simulink model "SMA_Wire_Controller"  (R2023b)
settings: Solver=FixedStepAuto  StartTime=0  StopTime=2  FixedStep=0.00001  RelTol=1e-5  EnableMultiTasking=on
values from neighbouring files (symbols this model uses):
  Da = 75.0e9    (= 75000000000)    [SMA_Initialize.m]
  Dm = 28.0e9    (= 28000000000)    [SMA_Initialize.m]
  epsR = 0.04    [SMA_Initialize.m]
  HeatCap = 837.3    [SMA_Initialize.m]
  HeatTransCoeff = 150    [SMA_Initialize.m]
  Inertia = 0.5*PullyMass*PullyRadius^2*0.001    (= 1e-08)    [SMA_Initialize.m]
  Length = 0.5    [SMA_Initialize.m]
  pa = 100*10^-8    (= 1e-06)    [SMA_Initialize.m]
  pm = 80*10^-8    (= 8e-07)    [SMA_Initialize.m]
  PullyRadius = 0.02    [SMA_Initialize.m]
  SectA = pi*(Diameter^2)/4    (= 3.14159265359e-08)    [SMA_Initialize.m]
  SurfArea = Diameter*Length*pi    (= 0.000314159265359)    [SMA_Initialize.m]
  TempAmb = 25    [SMA_Initialize.m]
  thetaT = 0    [SMA_Initialize.m]
  WireMass = (Density*pi*(Diameter^2)*Length)/4    (= 0.000101316363078)    [SMA_Initialize.m]
libraries: simulink x2
settings Model: Creator=Jack  LastModifiedBy=Jack
settings SolverCC: ZeroCrossControl=EnableAll  ZeroCrossAlgorithm=Adaptive
settings DebuggingCC: SignalInfNanChecking=error  ParameterPrecisionLossMsg=none
settings HardwareCC: ProdBitPerLong=64  ProdLargestAtomicFloat=Double  ProdHWDeviceType=AMD->Athlon 64

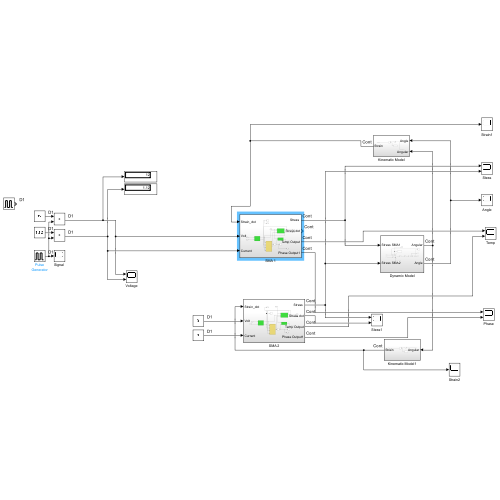
[thumbnail: Simulink's stored preview of the top-level diagram]
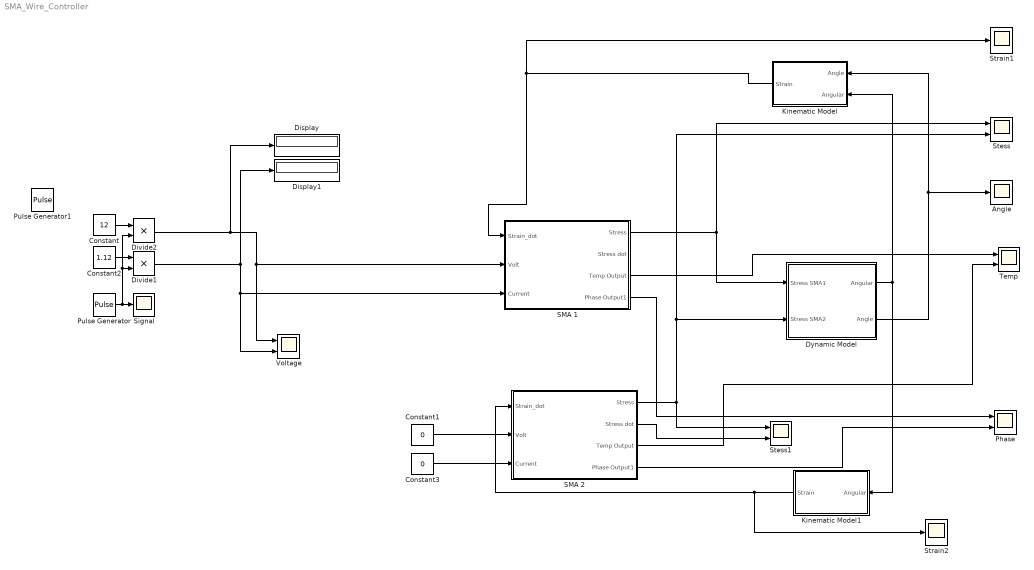
== system SMA_Wire_Controller ==
  Angle : Scope
  Constant : Constant  Value=12  SampleTime=0.00001
  Constant1 : Constant  Value=0  SampleTime=0.00001
  Constant2 : Constant  Value=1.12  SampleTime=0.00001
  Constant3 : Constant  Value=0  SampleTime=0.00001
  Display : Display
  Display1 : Display
  Divide1 : Product  Inputs=**
  Divide2 : Product  Inputs=**
  Dynamic Model : Subsystem
  Kinematic Model : Subsystem
  Kinematic Model1 : Subsystem
  Phase : Scope  NumInputPorts=2
  Pulse Generator : DiscretePulseGenerator  PulseType=Time based  Period=40  PulseWidth=1.5  PhaseDelay=0.25
  Pulse Generator1 : DiscretePulseGenerator  PulseType=Time based  Amplitude=0.5  Period=10  PulseWidth=5
  SMA 1 : Subsystem
  SMA 2 : Subsystem
  "Signal " : Scope
  Stess : Scope  NumInputPorts=2
  Stess1 : Scope  NumInputPorts=2
  Strain1 : Scope
  Strain2 : Scope
  Temp : Scope  NumInputPorts=2
  Voltage : Scope  NumInputPorts=2
  wires:
  Divide2/1 -> SMA 1/2(Volt), Voltage/1, Display/1
  Pulse Generator/1 -> Divide1/2, Divide2/2, "Signal "/1
  Divide1/1 -> Voltage/2, SMA 1/3(Current), Display1/1
  Dynamic Model/2(Angle) -> Kinematic Model/1(Angle), Angle/1
  Constant/1 -> Divide2/1
  Constant2/1 -> Divide1/1
  Kinematic Model/1(Strain) -> SMA 1/1(Strain_dot), Strain1/1
  Dynamic Model/1(Angular) -> Kinematic Model/2(Angular), Kinematic Model1/1(Angular)
  SMA 1/1("Stress ") -> Dynamic Model/1(Stress SMA1), Stess/1
  Kinematic Model1/1(Strain) -> Strain2/1, SMA 2/1(Strain_dot)
  SMA 2/1("Stress ") -> Stess1/1, Dynamic Model/2(Stress SMA2), Stess/2
  SMA 2/2(Stress dot) -> Stess1/2
  SMA 1/3(Temp Output) -> Temp/1
  SMA 2/3(Temp Output) -> Temp/2
  SMA 1/4(Phase Output1) -> Phase/1
  SMA 2/4(Phase Output1) -> Phase/2
  Constant1/1 -> SMA 2/2(Volt)
  Constant3/1 -> SMA 2/3(Current)

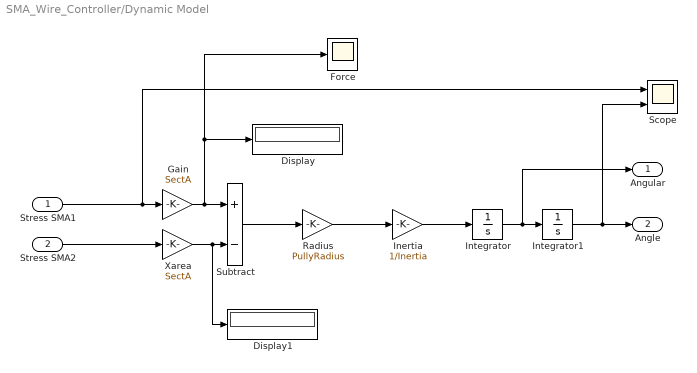
== system SMA_Wire_Controller/Dynamic Model ==
  Stress SMA1 : Inport
  Stress SMA2 : Inport  Port=2
  Display : Display
  Display1 : Display
  Force : Scope
  Gain : Gain  Gain=SectA
  Inertia : Gain  Gain=1/Inertia
  Integrator : Integrator
  Integrator1 : Integrator
  Radius : Gain  Gain=PullyRadius
  Scope : Scope  NumInputPorts=2
  Subtract : Sum  Inputs=+-
  Xarea : Gain  Gain=SectA  OutDataTypeStr=single
  Angular : Outport
  Angle : Outport  Port=2
  wires:
  Gain/1 -> Subtract/1, Display/1, Force/1
  Xarea/1 -> Display1/1, Subtract/2
  Subtract/1 -> Radius/1
  Radius/1 -> Inertia/1
  Inertia/1 -> Integrator/1
  Integrator/1 -> Angular/1, Integrator1/1
  Stress SMA1/1 -> Scope/1, Gain/1
  Stress SMA2/1 -> Xarea/1
  Integrator1/1 -> Angle/1, Scope/2

== system SMA_Wire_Controller/Kinematic Model ==
  Angle : Inport
  Angular : Inport  Port=2
  -r : Gain  Gain=-PullyRadius
  Constant : Constant  Value=Length  SampleTime=0.00001
  Divide : Product  Inputs=*/
  Strain : Outport
  wires:
  Constant/1 -> Divide/2
  -r/1 -> Divide/1
  Angle/1 -> -r/1
  Divide/1 -> Strain/1

== system SMA_Wire_Controller/Kinematic Model1 ==
  Angular : Inport
  -r : Gain  Gain=PullyRadius
  Constant : Constant  Value=Length  SampleTime=0.00001
  Divide : Product  Inputs=*/
  Strain : Outport
  wires:
  Constant/1 -> Divide/2
  -r/1 -> Divide/1
  Angular/1 -> -r/1
  Divide/1 -> Strain/1

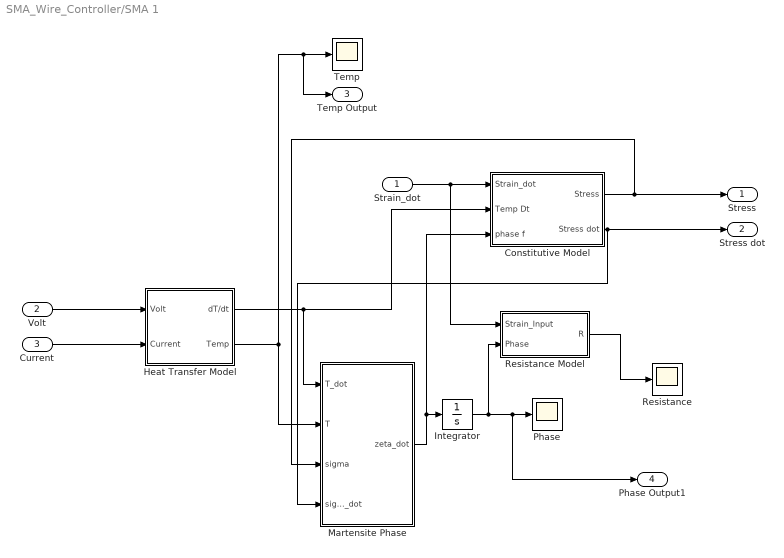
== system SMA_Wire_Controller/SMA 1 ==
  Strain_dot : Inport
  Volt : Inport  Port=2
  Current : Inport  Port=3
  Constitutive Model : Subsystem
  Heat Transfer Model : Subsystem
  Integrator : Integrator  InitialCondition=1
  "Martensite Phase " : Subsystem
  Phase : Scope
  Resistance : Scope
  Resistance Model : Subsystem
  Temp : Scope
  "Stress " : Outport
  Stress dot : Outport  Port=2
  Temp Output : Outport  Port=3
  Phase Output1 : Outport  Port=4
  wires:
  Current/1 -> Heat Transfer Model/2(Current)
  Resistance Model/1(R) -> Resistance/1
  Heat Transfer Model/1(dT/dt) -> "Martensite Phase "/1(T_dot), Constitutive Model/2(Temp Dt)
  "Martensite Phase "/1(zeta_dot) -> Constitutive Model/3(phase f), Integrator/1
  Volt/1 -> Heat Transfer Model/1(Volt)
  Strain_dot/1 -> Resistance Model/1(Strain_Input), Constitutive Model/1(Strain_dot)
  Heat Transfer Model/2(Temp) -> "Martensite Phase "/2(T), Temp Output/1, Temp/1
  Constitutive Model/1("Stress ") -> "Martensite Phase "/3(sigma), "Stress "/1
  Constitutive Model/2(Stress dot) -> "Martensite Phase "/4(sigma_dot), Stress dot/1
  Integrator/1 -> Resistance Model/2(Phase), Phase Output1/1, Phase/1

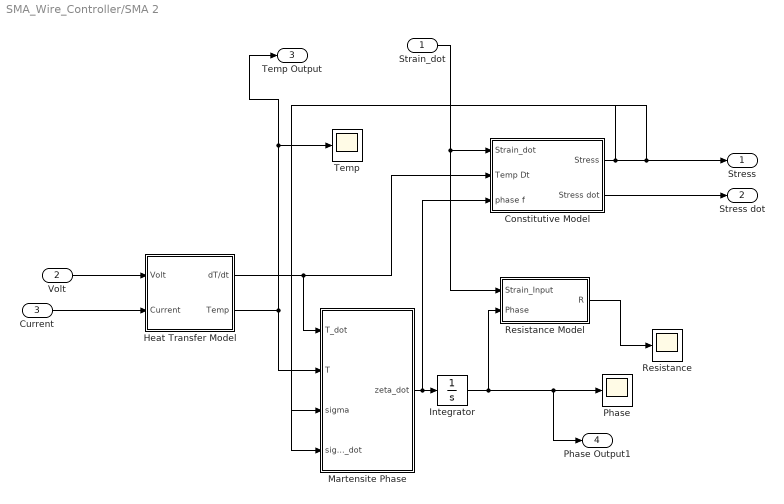
== system SMA_Wire_Controller/SMA 2 ==
  Strain_dot : Inport
  Volt : Inport  Port=2
  Current : Inport  Port=3
  Constitutive Model : Subsystem
  Heat Transfer Model : Subsystem
  Integrator : Integrator  InitialCondition=1
  "Martensite Phase " : Subsystem
  Phase : Scope
  Resistance : Scope
  Resistance Model : Subsystem
  Temp : Scope
  "Stress " : Outport
  Stress dot : Outport  Port=2
  Temp Output : Outport  Port=3
  Phase Output1 : Outport  Port=4
  wires:
  Current/1 -> Heat Transfer Model/2(Current)
  Resistance Model/1(R) -> Resistance/1
  Heat Transfer Model/1(dT/dt) -> "Martensite Phase "/1(T_dot), Constitutive Model/2(Temp Dt)
  Volt/1 -> Heat Transfer Model/1(Volt)
  Strain_dot/1 -> Resistance Model/1(Strain_Input), Constitutive Model/1(Strain_dot)
  Heat Transfer Model/2(Temp) -> "Martensite Phase "/2(T), Temp Output/1, Temp/1
  Constitutive Model/1("Stress ") -> "Martensite Phase "/3(sigma), "Martensite Phase "/4(sigma_dot), "Stress "/1
  Constitutive Model/2(Stress dot) -> Stress dot/1
  "Martensite Phase "/1(zeta_dot) -> Constitutive Model/3(phase f), Integrator/1
  Integrator/1 -> Resistance Model/2(Phase), Phase Output1/1, Phase/1

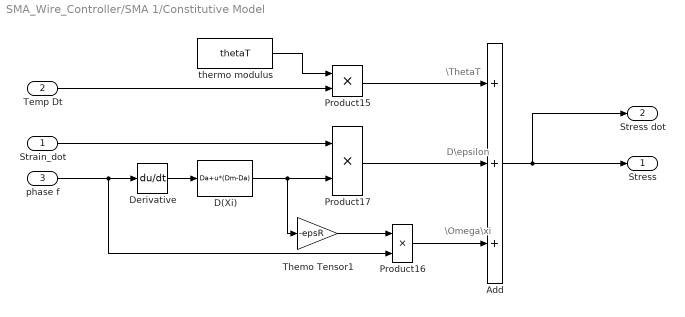
== system SMA_Wire_Controller/SMA 1/Constitutive Model ==
  note: \Omega\xi
  note: \ThetaT
  note: D\epsilon
  Strain_dot : Inport
  Temp Dt : Inport  Port=2
  phase f : Inport  Port=3
  Add : Sum  Inputs=+++
  D(Xi) : Fcn  Expr=Da+u*(Dm-Da)
  Derivative : Derivative
  Product15 : Product
  Product16 : Product
  Product17 : Product
  Themo Tensor1 : Gain  Gain=-epsR  SaturateOnIntegerOverflow=on  OutDataTypeStr=Inherit: Same as input  ParamDataTypeStr=Inherit: Same as input
  thermo modulus : Constant  Value=thetaT  SampleTime=0.00001
  "Stress " : Outport
  Stress dot : Outport  Port=2
  wires:
  Product15/1 -> Add/1
  Temp Dt/1 -> Product15/2
  thermo modulus/1 -> Product15/1
  D(Xi)/1 -> Product17/2, Themo Tensor1/1
  Themo Tensor1/1 -> Product16/1
  Add/1 -> "Stress "/1, Stress dot/1
  Product17/1 -> Add/2
  Product16/1 -> Add/3
  Strain_dot/1 -> Product17/1
  phase f/1 -> Derivative/1, Product16/2
  Derivative/1 -> D(Xi)/1

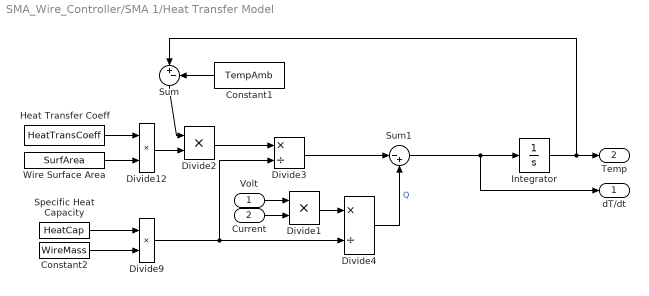
== system SMA_Wire_Controller/SMA 1/Heat Transfer Model ==
  Volt : Inport
  Current : Inport  Port=2
  Constant1 : Constant  Value=TempAmb  SampleTime=0.00001
  Constant2 : Constant  Value=WireMass  SampleTime=0.00001
  Divide{1..2,9,12} (4 alike) : Product  Inputs=**
  Divide3 : Product  Inputs=*/
  Divide4 : Product  Inputs=*/
  Heat Transfer Coeff : Constant  Value=HeatTransCoeff  SampleTime=0.00001
  Integrator : Integrator  InitialCondition=TempAmb
  Specific Heat Capacity : Constant  Value=HeatCap  SampleTime=0.00001
  Sum : Sum  Inputs=|+-
  Sum1 : Sum  Inputs=|-+
  Wire Surface Area : Constant  Value=SurfArea  SampleTime=0.00001
  dT/dt : Outport
  Temp : Outport  Port=2
  wires:
  Divide4/1 -> Sum1/2  "Q"
  Integrator/1 -> Temp/1, Sum/1
  Divide2/1 -> Divide3/1
  Heat Transfer Coeff/1 -> Divide12/1
  Divide9/1 -> Divide4/2, Divide3/2
  Constant1/1 -> Sum/2
  Wire Surface Area/1 -> Divide12/2
  Volt/1 -> Divide1/1
  Current/1 -> Divide1/2
  Divide12/1 -> Divide2/2
  Specific Heat Capacity/1 -> Divide9/1
  Divide1/1 -> Divide4/1
  Divide3/1 -> Sum1/1
  Sum/1 -> Divide2/1
  Sum1/1 -> dT/dt/1, Integrator/1
  Constant2/1 -> Divide9/2

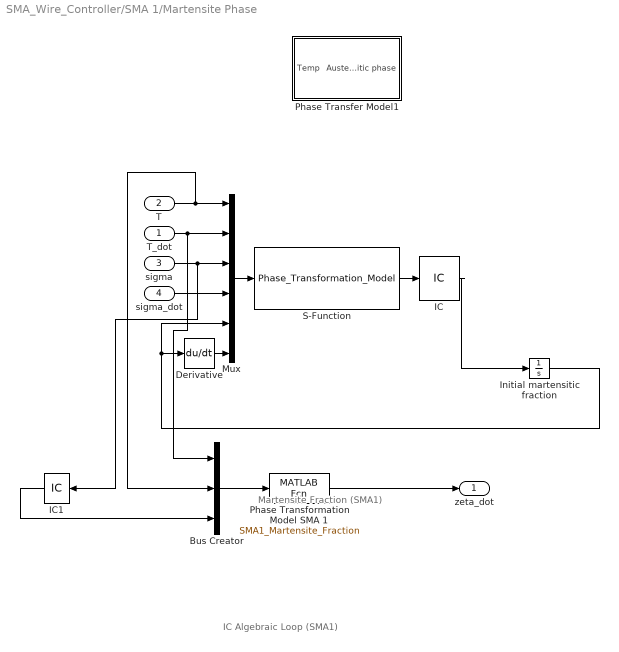
== system SMA_Wire_Controller/SMA 1/Martensite Phase  ==
  note: Martensite
      | Fraction (SMA1)
  note: IC Algebraic
      | Loop (SMA1)
  T_dot : Inport
  T : Inport  Port=2
  sigma : Inport  Port=3
  sigma_dot : Inport  Port=4
  Bus Creator : BusCreator  DialogController=Simulink.DDGSource_Bus  Inputs=3
  Derivative : Derivative
  IC : InitialCondition  Value=0
  IC1 : InitialCondition  Value=0
  Initial martensitic fraction : Integrator  InitialCondition=1  UpperSaturationLimit=1  LowerSaturationLimit=0
  Mux : Mux  Inputs=6
  Phase Transfer Model1 : Subsystem
  Phase Transformation Model SMA 1 : MATLABFcn  MATLABFcn=SMA1_Martensite_Fraction  OutputDimensions=1
  S-Function : S-Function  FunctionName=Phase_Transformation_Model  SFunctionDeploymentMode=off  EnableBusSupport=off
  zeta_dot : Outport
  wires:
  Initial martensitic fraction/1 -> Derivative/1, Mux/5
  Derivative/1 -> Mux/6
  S-Function/1 -> IC/1
  sigma_dot/1 -> Mux/4
  Mux/1 -> S-Function/1
  T/1 -> Bus Creator/2, Mux/1
  sigma/1 -> IC1/1, Mux/3
  T_dot/1 -> Bus Creator/1, Mux/2
  IC/1 -> Initial martensitic fraction/1
  IC1/1 -> Bus Creator/3
  Phase Transformation Model SMA 1/1 -> zeta_dot/1
  Bus Creator/1 -> Phase Transformation Model SMA 1/1

== system SMA_Wire_Controller/SMA 1/Resistance Model ==
  Strain_Input : Inport
  Phase : Inport  Port=2
  Constant : Constant
  Product : Product
  Product1 : Product
  Ra : Subsystem
  Rm : Subsystem
  Scope : Scope  NumInputPorts=2
  Subtract : Sum  Inputs=+-
  Sum : Sum  Inputs=|++
  R : Outport
  wires:
  Rm/1(Rm) -> Product/1
  Sum/1 -> R/1
  Product/1 -> Scope/1, Sum/1
  Constant/1 -> Subtract/1
  Phase/1 -> Subtract/2, Product/2
  Subtract/1 -> Product1/1
  Ra/1(Ra) -> Product1/2
  Product1/1 -> Sum/2, Scope/2
  Strain_Input/1 -> Ra/1(Strain), Rm/1(Strain)

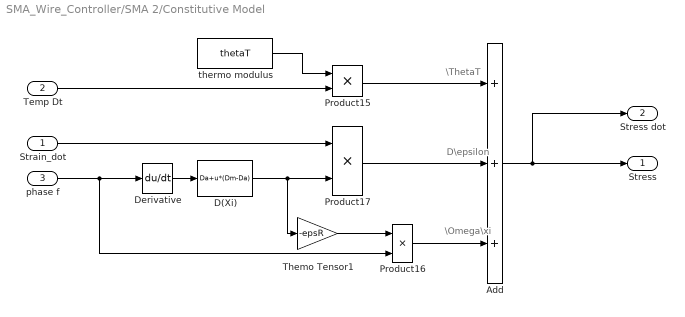
== system SMA_Wire_Controller/SMA 2/Constitutive Model ==
  note: \Omega\xi
  note: \ThetaT
  note: D\epsilon
  Strain_dot : Inport
  Temp Dt : Inport  Port=2
  phase f : Inport  Port=3
  Add : Sum  Inputs=+++
  D(Xi) : Fcn  Expr=Da+u*(Dm-Da)
  Derivative : Derivative
  Product15 : Product
  Product16 : Product
  Product17 : Product
  Themo Tensor1 : Gain  Gain=-epsR  SaturateOnIntegerOverflow=on  OutDataTypeStr=Inherit: Same as input  ParamDataTypeStr=Inherit: Same as input
  thermo modulus : Constant  Value=thetaT  SampleTime=0.00001
  "Stress " : Outport
  Stress dot : Outport  Port=2
  wires:
  Product15/1 -> Add/1
  Temp Dt/1 -> Product15/2
  thermo modulus/1 -> Product15/1
  D(Xi)/1 -> Product17/2, Themo Tensor1/1
  Themo Tensor1/1 -> Product16/1
  Add/1 -> "Stress "/1, Stress dot/1
  Product17/1 -> Add/2
  Product16/1 -> Add/3
  Strain_dot/1 -> Product17/1
  phase f/1 -> Derivative/1, Product16/2
  Derivative/1 -> D(Xi)/1

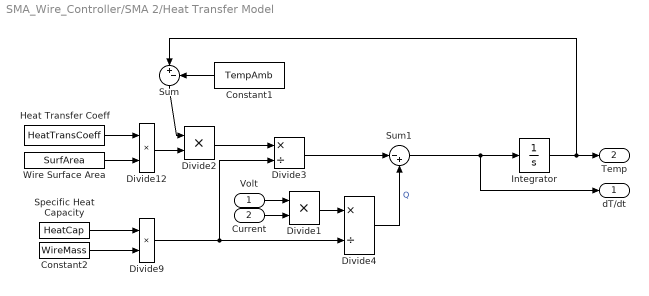
== system SMA_Wire_Controller/SMA 2/Heat Transfer Model ==
  Volt : Inport
  Current : Inport  Port=2
  Constant1 : Constant  Value=TempAmb  SampleTime=0.00001
  Constant2 : Constant  Value=WireMass  SampleTime=0.00001
  Divide{1..2,9,12} (4 alike) : Product  Inputs=**
  Divide3 : Product  Inputs=*/
  Divide4 : Product  Inputs=*/
  Heat Transfer Coeff : Constant  Value=HeatTransCoeff  SampleTime=0.00001
  Integrator : Integrator  InitialCondition=TempAmb
  Specific Heat Capacity : Constant  Value=HeatCap  SampleTime=0.00001
  Sum : Sum  Inputs=|+-
  Sum1 : Sum  Inputs=|-+
  Wire Surface Area : Constant  Value=SurfArea  SampleTime=0.00001
  dT/dt : Outport
  Temp : Outport  Port=2
  wires:
  Divide4/1 -> Sum1/2  "Q"
  Integrator/1 -> Temp/1, Sum/1
  Divide2/1 -> Divide3/1
  Heat Transfer Coeff/1 -> Divide12/1
  Divide9/1 -> Divide4/2, Divide3/2
  Constant1/1 -> Sum/2
  Wire Surface Area/1 -> Divide12/2
  Volt/1 -> Divide1/1
  Current/1 -> Divide1/2
  Divide12/1 -> Divide2/2
  Specific Heat Capacity/1 -> Divide9/1
  Divide1/1 -> Divide4/1
  Divide3/1 -> Sum1/1
  Sum/1 -> Divide2/1
  Sum1/1 -> dT/dt/1, Integrator/1
  Constant2/1 -> Divide9/2

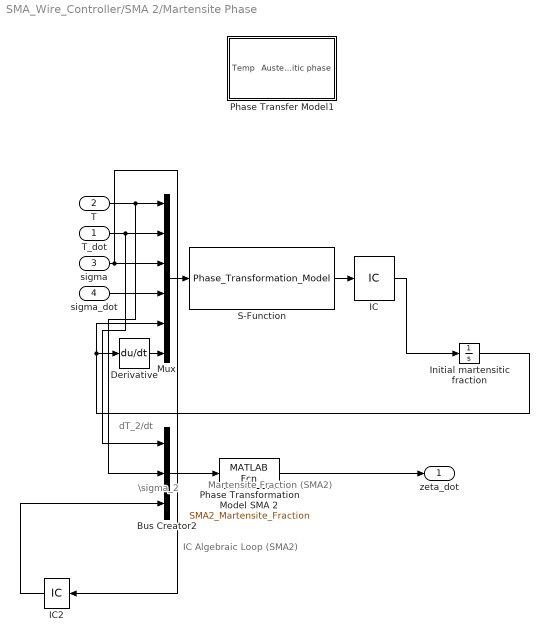
== system SMA_Wire_Controller/SMA 2/Martensite Phase  ==
  note: \sigma_2
  note: IC Algebraic
      | Loop (SMA2)
  note: Martensite
      | Fraction (SMA2)
  note: dT_2/dt
  T_dot : Inport
  T : Inport  Port=2
  sigma : Inport  Port=3
  sigma_dot : Inport  Port=4
  Bus Creator2 : BusCreator  DialogController=Simulink.DDGSource_Bus  Inputs=3
  Derivative : Derivative
  IC : InitialCondition  Value=0
  IC2 : InitialCondition  Value=0
  Initial martensitic fraction : Integrator  InitialCondition=1  UpperSaturationLimit=1  LowerSaturationLimit=0
  Mux : Mux  Inputs=6
  Phase Transfer Model1 : Subsystem
  Phase Transformation Model SMA 2 : MATLABFcn  MATLABFcn=SMA2_Martensite_Fraction  OutputDimensions=1
  S-Function : S-Function  FunctionName=Phase_Transformation_Model  SFunctionDeploymentMode=off  EnableBusSupport=off
  zeta_dot : Outport
  wires:
  Initial martensitic fraction/1 -> Derivative/1, Mux/5
  Derivative/1 -> Mux/6
  S-Function/1 -> IC/1
  sigma_dot/1 -> Mux/4
  Mux/1 -> S-Function/1
  T_dot/1 -> Bus Creator2/1, Mux/2
  IC/1 -> Initial martensitic fraction/1
  Phase Transformation Model SMA 2/1 -> zeta_dot/1
  Bus Creator2/1 -> Phase Transformation Model SMA 2/1
  T/1 -> Bus Creator2/2, Mux/1
  IC2/1 -> Bus Creator2/3
  sigma/1 -> Mux/3, IC2/1

== system SMA_Wire_Controller/SMA 2/Resistance Model ==
  Strain_Input : Inport
  Phase : Inport  Port=2
  Constant : Constant
  Product : Product
  Product1 : Product
  Ra : Subsystem
  Rm : Subsystem
  Scope : Scope  NumInputPorts=2
  Subtract : Sum  Inputs=+-
  Sum : Sum  Inputs=|++
  R : Outport
  wires:
  Rm/1(Rm) -> Product/1
  Sum/1 -> R/1
  Product/1 -> Scope/1, Sum/1
  Constant/1 -> Subtract/1
  Phase/1 -> Subtract/2, Product/2
  Subtract/1 -> Product1/1
  Ra/1(Ra) -> Product1/2
  Product1/1 -> Sum/2, Scope/2
  Strain_Input/1 -> Ra/1(Strain), Rm/1(Strain)

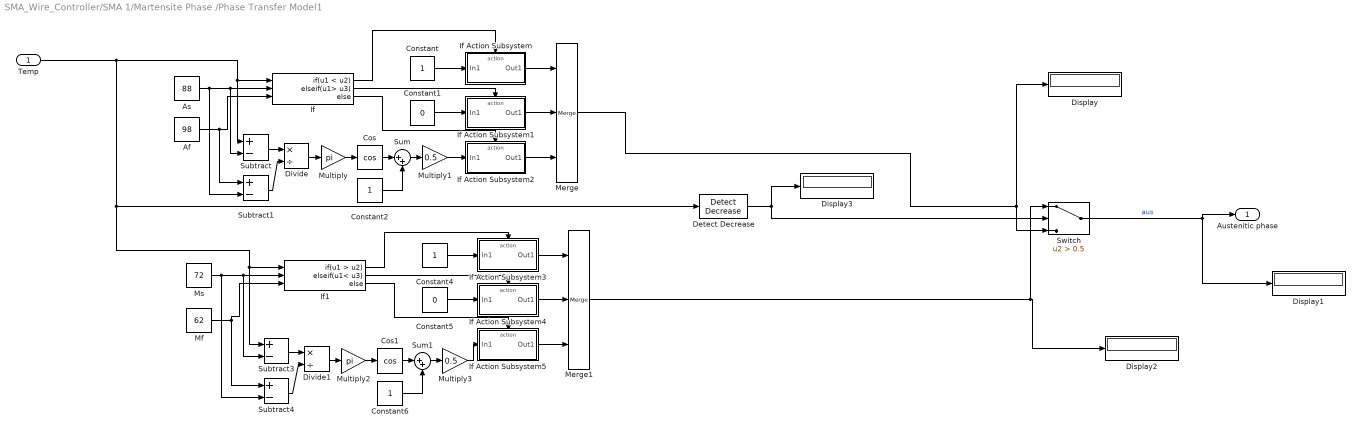
== system SMA_Wire_Controller/SMA 1/Martensite Phase /Phase Transfer Model1 ==
  Temp : Inport
  Af : Constant  Value=98
  As : Constant  Value=88
  Constant{,2,4,6} (4 alike) : Constant
  Constant1 : Constant  Value=0
  Constant5 : Constant  Value=0
  Cos : Trigonometry  Operator=cos
  Cos1 : Trigonometry  Operator=cos
  Detect Decrease : simulink/Logic and Bit Operations/Detect Decrease  vinit=0  OutDataTypeStr=uint8
  Display{,1..3} (4 alike) : Display
  Divide : Product  Inputs=*/
  Divide1 : Product  Inputs=*/
  If : If  NumInputs=3  IfExpression=u1 < u2  ElseIfExpressions=u1> u3
  If Action Subsystem : Subsystem  TreatAsAtomicUnit=on
  If Action Subsystem1 : Subsystem  TreatAsAtomicUnit=on
  If Action Subsystem2 : Subsystem  TreatAsAtomicUnit=on
  If Action Subsystem3 : Subsystem  TreatAsAtomicUnit=on
  If Action Subsystem4 : Subsystem  TreatAsAtomicUnit=on
  If Action Subsystem5 : Subsystem  TreatAsAtomicUnit=on
  If1 : If  NumInputs=3  IfExpression=u1 > u2  ElseIfExpressions=u1< u3
  Merge : Merge  Inputs=3
  Merge1 : Merge  Inputs=3
  Mf : Constant  Value=62
  Ms : Constant  Value=72
  Multiply : Gain  Gain=pi
  Multiply1 : Gain  Gain=0.5
  Multiply2 : Gain  Gain=pi
  Multiply3 : Gain  Gain=0.5
  Subtract{,1,3..4} (4 alike) : Sum  Inputs=+-
  Sum : Sum  Inputs=|++
  Sum1 : Sum  Inputs=|++
  Switch : Switch  Criteria=u2 > Threshold  Threshold=0.5  SaturateOnIntegerOverflow=off  InputSameDT=off
  "Austenitic phase " : Outport
  wires:
  As/1 -> Subtract1/2, Subtract/2, If/2
  Af/1 -> Subtract1/1, If/3
  If/1 -> If Action Subsystem/Action
  If/2 -> If Action Subsystem1/Action
  Constant/1 -> If Action Subsystem/1(In1)
  Constant1/1 -> If Action Subsystem1/1(In1)
  If/3 -> If Action Subsystem2/Action
  If Action Subsystem/1(Out1) -> Merge/1
  If Action Subsystem1/1(Out1) -> Merge/2
  If Action Subsystem2/1(Out1) -> Merge/3
  Subtract/1 -> Divide/1
  Subtract1/1 -> Divide/2
  Divide/1 -> Multiply/1
  Multiply/1 -> Cos/1
  Cos/1 -> Sum/1
  Constant2/1 -> Sum/2
  Sum/1 -> Multiply1/1
  Multiply1/1 -> If Action Subsystem2/1(In1)
  Divide1/1 -> Multiply2/1
  If Action Subsystem4/1(Out1) -> Merge1/2
  Multiply2/1 -> Cos1/1
  Mf/1 -> If1/3, Subtract4/1
  Cos1/1 -> Sum1/1
  Subtract3/1 -> Divide1/1
  Subtract4/1 -> Divide1/2
  Sum1/1 -> Multiply3/1
  Constant4/1 -> If Action Subsystem3/1(In1)
  If1/1 -> If Action Subsystem3/Action
  If1/3 -> If Action Subsystem5/Action
  If1/2 -> If Action Subsystem4/Action
  Constant5/1 -> If Action Subsystem4/1(In1)
  Ms/1 -> Subtract4/2, Subtract3/2, If1/2
  Constant6/1 -> Sum1/2
  Multiply3/1 -> If Action Subsystem5/1(In1)
  If Action Subsystem5/1(Out1) -> Merge1/3
  If Action Subsystem3/1(Out1) -> Merge1/1
  Temp/1 -> Detect Decrease/1, Subtract3/1, If1/1, Subtract/1, If/1
  Detect Decrease/1 -> Switch/2, Display3/1
  Merge1/1 -> Switch/1, Display2/1
  Merge/1 -> Switch/3, Display/1
  Switch/1 -> "Austenitic phase "/1, Display1/1  "aus"

== system SMA_Wire_Controller/SMA 1/Resistance Model/Ra ==
  Strain : Inport
  Divide : Product  Inputs=*/
  Product2 : Product
  Sum1 : Sum  Inputs=|++
  p_m : Constant  Value=pa
  p_m1 : Constant  Value=Length
  p_m2 : Constant  Value=SectA
  Ra : Outport
  wires:
  p_m1/1 -> Sum1/1
  Strain/1 -> Sum1/2
  p_m/1 -> Product2/1
  Sum1/1 -> Product2/2
  p_m2/1 -> Divide/2
  Product2/1 -> Divide/1
  Divide/1 -> Ra/1

== system SMA_Wire_Controller/SMA 1/Resistance Model/Rm ==
  Strain : Inport
  Divide : Product  Inputs=*/
  Product2 : Product
  Sum1 : Sum  Inputs=|++
  p_m : Constant  Value=pm
  p_m1 : Constant  Value=Length
  p_m2 : Constant  Value=SectA
  Rm : Outport
  wires:
  p_m1/1 -> Sum1/1
  Strain/1 -> Sum1/2
  p_m/1 -> Product2/1
  Sum1/1 -> Product2/2
  p_m2/1 -> Divide/2
  Product2/1 -> Divide/1
  Divide/1 -> Rm/1

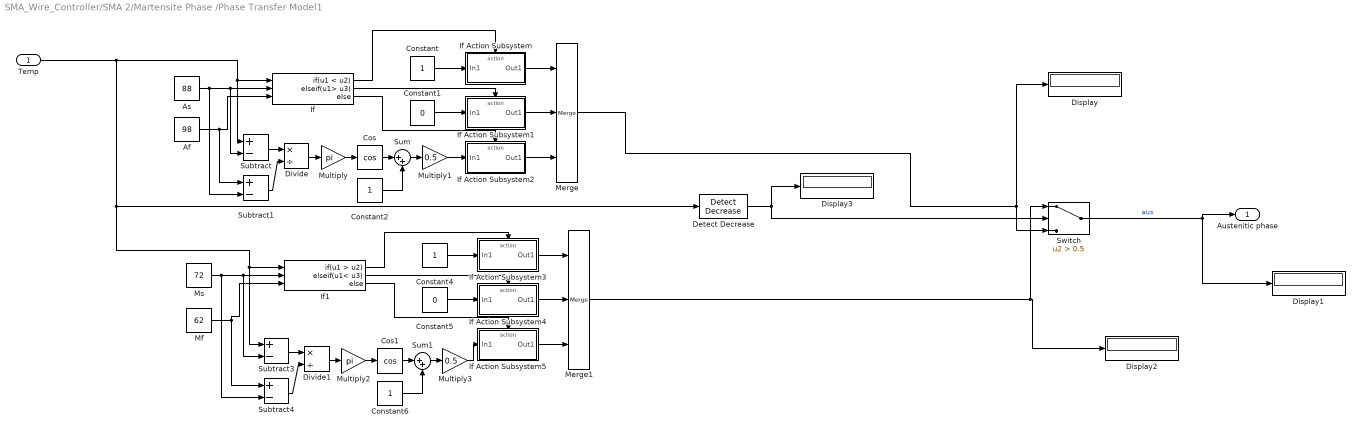
== system SMA_Wire_Controller/SMA 2/Martensite Phase /Phase Transfer Model1 ==
  Temp : Inport
  Af : Constant  Value=98
  As : Constant  Value=88
  Constant{,2,4,6} (4 alike) : Constant
  Constant1 : Constant  Value=0
  Constant5 : Constant  Value=0
  Cos : Trigonometry  Operator=cos
  Cos1 : Trigonometry  Operator=cos
  Detect Decrease : simulink/Logic and Bit Operations/Detect Decrease  vinit=0  OutDataTypeStr=uint8
  Display{,1..3} (4 alike) : Display
  Divide : Product  Inputs=*/
  Divide1 : Product  Inputs=*/
  If : If  NumInputs=3  IfExpression=u1 < u2  ElseIfExpressions=u1> u3
  If Action Subsystem : Subsystem  TreatAsAtomicUnit=on
  If Action Subsystem1 : Subsystem  TreatAsAtomicUnit=on
  If Action Subsystem2 : Subsystem  TreatAsAtomicUnit=on
  If Action Subsystem3 : Subsystem  TreatAsAtomicUnit=on
  If Action Subsystem4 : Subsystem  TreatAsAtomicUnit=on
  If Action Subsystem5 : Subsystem  TreatAsAtomicUnit=on
  If1 : If  NumInputs=3  IfExpression=u1 > u2  ElseIfExpressions=u1< u3
  Merge : Merge  Inputs=3
  Merge1 : Merge  Inputs=3
  Mf : Constant  Value=62
  Ms : Constant  Value=72
  Multiply : Gain  Gain=pi
  Multiply1 : Gain  Gain=0.5
  Multiply2 : Gain  Gain=pi
  Multiply3 : Gain  Gain=0.5
  Subtract{,1,3..4} (4 alike) : Sum  Inputs=+-
  Sum : Sum  Inputs=|++
  Sum1 : Sum  Inputs=|++
  Switch : Switch  Criteria=u2 > Threshold  Threshold=0.5  SaturateOnIntegerOverflow=off  InputSameDT=off
  "Austenitic phase " : Outport
  wires:
  As/1 -> Subtract1/2, Subtract/2, If/2
  Af/1 -> Subtract1/1, If/3
  If/1 -> If Action Subsystem/Action
  If/2 -> If Action Subsystem1/Action
  Constant/1 -> If Action Subsystem/1(In1)
  Constant1/1 -> If Action Subsystem1/1(In1)
  If/3 -> If Action Subsystem2/Action
  If Action Subsystem/1(Out1) -> Merge/1
  If Action Subsystem1/1(Out1) -> Merge/2
  If Action Subsystem2/1(Out1) -> Merge/3
  Subtract/1 -> Divide/1
  Subtract1/1 -> Divide/2
  Divide/1 -> Multiply/1
  Multiply/1 -> Cos/1
  Cos/1 -> Sum/1
  Constant2/1 -> Sum/2
  Sum/1 -> Multiply1/1
  Multiply1/1 -> If Action Subsystem2/1(In1)
  Divide1/1 -> Multiply2/1
  If Action Subsystem4/1(Out1) -> Merge1/2
  Multiply2/1 -> Cos1/1
  Mf/1 -> If1/3, Subtract4/1
  Cos1/1 -> Sum1/1
  Subtract3/1 -> Divide1/1
  Subtract4/1 -> Divide1/2
  Sum1/1 -> Multiply3/1
  Constant4/1 -> If Action Subsystem3/1(In1)
  If1/1 -> If Action Subsystem3/Action
  If1/3 -> If Action Subsystem5/Action
  If1/2 -> If Action Subsystem4/Action
  Constant5/1 -> If Action Subsystem4/1(In1)
  Ms/1 -> Subtract4/2, Subtract3/2, If1/2
  Constant6/1 -> Sum1/2
  Multiply3/1 -> If Action Subsystem5/1(In1)
  If Action Subsystem5/1(Out1) -> Merge1/3
  If Action Subsystem3/1(Out1) -> Merge1/1
  Temp/1 -> Detect Decrease/1, Subtract3/1, If1/1, Subtract/1, If/1
  Detect Decrease/1 -> Switch/2, Display3/1
  Merge1/1 -> Switch/1, Display2/1
  Merge/1 -> Switch/3, Display/1
  Switch/1 -> "Austenitic phase "/1, Display1/1  "aus"

== system SMA_Wire_Controller/SMA 2/Resistance Model/Ra ==
  Strain : Inport
  Divide : Product  Inputs=*/
  Product2 : Product
  Sum1 : Sum  Inputs=|++
  p_m : Constant  Value=pa
  p_m1 : Constant  Value=Length
  p_m2 : Constant  Value=SectA
  Ra : Outport
  wires:
  p_m1/1 -> Sum1/1
  Strain/1 -> Sum1/2
  p_m/1 -> Product2/1
  Sum1/1 -> Product2/2
  p_m2/1 -> Divide/2
  Product2/1 -> Divide/1
  Divide/1 -> Ra/1

== system SMA_Wire_Controller/SMA 2/Resistance Model/Rm ==
  Strain : Inport
  Divide : Product  Inputs=*/
  Product2 : Product
  Sum1 : Sum  Inputs=|++
  p_m : Constant  Value=pm
  p_m1 : Constant  Value=Length
  p_m2 : Constant  Value=SectA
  Rm : Outport
  wires:
  p_m1/1 -> Sum1/1
  Strain/1 -> Sum1/2
  p_m/1 -> Product2/1
  Sum1/1 -> Product2/2
  p_m2/1 -> Divide/2
  Product2/1 -> Divide/1
  Divide/1 -> Rm/1

== system SMA_Wire_Controller/SMA 1/Martensite Phase /Phase Transfer Model1/If Action Subsystem ==
  In1 : Inport
  Action Port : ActionPort  ActionPortLabel=if(u1 < u2)
  Out1 : Outport
  wires:
  In1/1 -> Out1/1

== system SMA_Wire_Controller/SMA 1/Martensite Phase /Phase Transfer Model1/If Action Subsystem1 ==
  In1 : Inport
  Action Port : ActionPort  ActionPortLabel=elseif(u1> u3)
  Out1 : Outport
  wires:
  In1/1 -> Out1/1

== system SMA_Wire_Controller/SMA 1/Martensite Phase /Phase Transfer Model1/If Action Subsystem2 ==
  In1 : Inport
  Action Port : ActionPort  ActionPortLabel=else
  Out1 : Outport
  wires:
  In1/1 -> Out1/1

== system SMA_Wire_Controller/SMA 1/Martensite Phase /Phase Transfer Model1/If Action Subsystem3 ==
  In1 : Inport
  Action Port : ActionPort  ActionPortLabel=if(u1 > u2)
  Out1 : Outport
  wires:
  In1/1 -> Out1/1

== system SMA_Wire_Controller/SMA 1/Martensite Phase /Phase Transfer Model1/If Action Subsystem4 ==
  In1 : Inport
  Action Port : ActionPort  ActionPortLabel=elseif(u1< u3)
  Out1 : Outport
  wires:
  In1/1 -> Out1/1

== system SMA_Wire_Controller/SMA 1/Martensite Phase /Phase Transfer Model1/If Action Subsystem5 ==
  In1 : Inport
  Action Port : ActionPort  ActionPortLabel=else
  Out1 : Outport
  wires:
  In1/1 -> Out1/1

== system SMA_Wire_Controller/SMA 2/Martensite Phase /Phase Transfer Model1/If Action Subsystem ==
  In1 : Inport
  Action Port : ActionPort  ActionPortLabel=if(u1 < u2)
  Out1 : Outport
  wires:
  In1/1 -> Out1/1

== system SMA_Wire_Controller/SMA 2/Martensite Phase /Phase Transfer Model1/If Action Subsystem1 ==
  In1 : Inport
  Action Port : ActionPort  ActionPortLabel=elseif(u1> u3)
  Out1 : Outport
  wires:
  In1/1 -> Out1/1

== system SMA_Wire_Controller/SMA 2/Martensite Phase /Phase Transfer Model1/If Action Subsystem2 ==
  In1 : Inport
  Action Port : ActionPort  ActionPortLabel=else
  Out1 : Outport
  wires:
  In1/1 -> Out1/1

== system SMA_Wire_Controller/SMA 2/Martensite Phase /Phase Transfer Model1/If Action Subsystem3 ==
  In1 : Inport
  Action Port : ActionPort  ActionPortLabel=if(u1 > u2)
  Out1 : Outport
  wires:
  In1/1 -> Out1/1

== system SMA_Wire_Controller/SMA 2/Martensite Phase /Phase Transfer Model1/If Action Subsystem4 ==
  In1 : Inport
  Action Port : ActionPort  ActionPortLabel=elseif(u1< u3)
  Out1 : Outport
  wires:
  In1/1 -> Out1/1

== system SMA_Wire_Controller/SMA 2/Martensite Phase /Phase Transfer Model1/If Action Subsystem5 ==
  In1 : Inport
  Action Port : ActionPort  ActionPortLabel=else
  Out1 : Outport
  wires:
  In1/1 -> Out1/1
